simulink model "pitch_loop"  (Simulink 8.0)
settings: Solver=ode45  StartTime=0.0  StopTime=30  RelTol=1e-3
values from neighbouring files (symbols this model uses):
  a_theta1 = den(2)    [computeGains.m]
  a_theta2 = den(3)    [computeGains.m]
  a_theta3 = num(3)    [computeGains.m]
  delta_e_max = 45*pi/180    (= 0.785398163397)    [computeGains.m]
  theta_max = 15*pi/180    (= 0.261799387799)    [computeGains.m]
undefined symbols (not defined in the file or in its folder): P
settings Model: Creator=beard  LastModifiedBy=tmclain
settings DataIOCC: SignalLoggingSaveFormat=ModelDataLogs
settings DebuggingCC: FcnCallInpInsideContextMsg=UseLocalSettings  StrictBusMsg=Warning
settings GRTTargetCC: CombineOutputUpdateFcns=off  GRTInterface=on

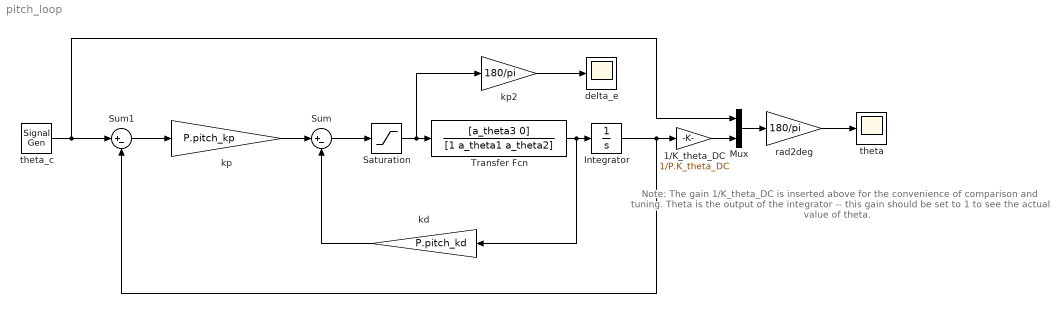
== system pitch_loop ==
  note: Note: The gain 1/K_theta_DC is inserted above for the convenience
      | of comparison and tuning. Theta is the output of the integrator -- this gain
      | should be set to 1 to see the actual value of theta.
  1/K_theta_DC : Gain  Gain=1/P.K_theta_DC
  Integrator : Integrator
  Mux : Mux  Inputs=2
  Saturation : Saturate  UpperLimit=delta_e_max  LowerLimit=-delta_e_max
  Sum : Sum  Inputs=|+-
  Sum1 : Sum  Inputs=|+-
  Transfer Fcn : TransferFcn  Numerator=[a_theta3 0]  Denominator=[1 a_theta1 a_theta2]
  delta_e : Scope
      settings: TimeRange=30  YMin=-100  YMax=100
  kd : Gain  Gain=P.pitch_kd
  kp : Gain  Gain=P.pitch_kp
  kp2 : Gain  Gain=180/pi
  rad2deg : Gain  Gain=180/pi
  theta : Scope
      settings: TimeRange=30  YMin=-15  YMax=15
  theta_c : SignalGenerator  WaveForm=square  Amplitude=theta_max  Frequency=.05
  wires:
  Transfer Fcn/1 -> Integrator/1, kd/1
  Saturation/1 -> Transfer Fcn/1, kp2/1
  Sum/1 -> Saturation/1
  Sum1/1 -> kp/1
  Integrator/1 -> Sum1/2, 1/K_theta_DC/1
  theta_c/1 -> Sum1/1, Mux/1
  rad2deg/1 -> theta/1
  Mux/1 -> rad2deg/1
  kp2/1 -> delta_e/1
  kp/1 -> Sum/1
  kd/1 -> Sum/2
  1/K_theta_DC/1 -> Mux/2
